simulink model "Modelo_estados_lazo_abierto"  (R2021a)
settings: Solver=VariableStepAuto  StartTime=0.0  StopTime=5  FixedStep=0.001  RelTol=1e-3
settings Model: Creator=faust  LastModifiedBy=faust

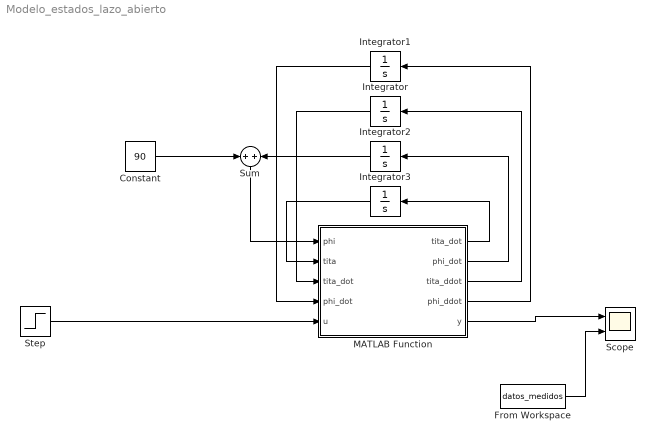
== system Modelo_estados_lazo_abierto ==
  Constant : Constant  Value=90
  From Workspace : FromWorkspace  VariableName=datos_medidos  SampleTime=0.01
  Integrator{,1..3} (4 alike) : Integrator
  MATLAB Function : MATLAB Function  TreatAsAtomicUnit=on
  Scope : Scope  NumInputPorts=2
  Step : Step  Time=0.04  Before=90  After=120  SampleTime=0.01
  Sum : Sum  Inputs=+|+
  wires:
  MATLAB Function/3(tita_ddot) -> Integrator/1
  Integrator/1 -> MATLAB Function/3("tita_dot ")
  MATLAB Function/5(y) -> Scope/1
  MATLAB Function/4(phi_ddot) -> Integrator1/1
  Integrator1/1 -> MATLAB Function/4("phi_dot ")
  MATLAB Function/1(tita_dot) -> Integrator3/1
  MATLAB Function/2(phi_dot) -> Integrator2/1
  Integrator3/1 -> MATLAB Function/2(tita)
  Constant/1 -> Sum/1
  Sum/1 -> MATLAB Function/1(phi)
  Integrator2/1 -> Sum/2
  Step/1 -> MATLAB Function/5(u)
  From Workspace/1 -> Scope/2

== matlab function Modelo_estados_lazo_abierto/MATLAB Function ==
  data: tita_dot output; phi_dot output; phi input; tita input; tita_dot input; phi_dot input; tita_ddot output; phi_ddot output; u input; y output
function [tita_dot,phi_dot,tita_ddot,phi_ddot,y] = fcn(phi, tita, tita_dot,phi_dot,u)

a = 0.7;
b = 2.613;
c = 65;
d = 292.2;
e = 30.67;
f = d;

phi_ddot = d * u - e * phi_dot - f * phi;
tita_ddot = phi_ddot * a - b * tita_dot - c * tita;

y = tita;
